simulink model "Nov12_RateModulated"  (R2019b)
settings: Solver=FixedStepAuto  StartTime=0.0  StopTime=10.0  FixedStep=1E-3  RelTol=1e-3
undefined symbols (not defined in the file): D0, D1, D10, D11, D12, D13, D2, D3, D4, D5, D6, D7, D8, D9, PTA0, PTA1, PTA2, PTB23, PTB9, PTC16, PTC17, PTC2, PTC3, PTC4, PTD0, PTD1, PTD2, PTD3
libraries: frdmk64flib x18
settings Model: PacingRate=0.100000  ExtModeTrigDuration=5  Creator=scotts24  LastModifiedBy=scotts24
settings DataIOCC: ReturnWorkspaceOutputs=off
settings OptimizationCC: PassReuseOutputArgsThreshold=0  MaxStackSize=64
settings DebuggingCC: ParameterTunabilityLossMsg=error  ArithmeticOperatorsInVariantConditions=warning
settings HardwareCC: ProdBitPerPointer=32  ProdBitPerSizeT=32  ProdBitPerPtrDiffT=32  ProdLargestAtomicInteger=Long  ProdLargestAtomicFloat=Double  ProdWordSize=32  ProdHWDeviceType=ARM Compatible->ARM Cortex  UseEmbeddedCoderFeatures=off
settings SFSimCC: SimUseLocalCustomCode=off  MATLABDynamicMemAlloc=off  CustomCodeUndefinedFunction=UseInterfaceOnly
settings RTWCC: SystemTargetFile=ert.tlc  HardwareBoard=NXP FRDM-K64F  TLCOptions="-aInlineSetEventsForThisBaseRateFcn=TLC_FALSE -aSuppressMultiTaskScheduler=TLC_FALSE  -aRateBasedStepFcn=0"  TemplateMakefile=ert_default_tmf  GenerateReport=on  RTWUseLocalCustomCode=off  Toolchain=GNU Tools for ARM Embedded Processors  LaunchReport=on
settings CodeAppCC: ForceParamTrailComments=on  OperatorAnnotations=on
settings ERTTargetCC: ERTCustomFileBanners=off  SupportContinuousTime=on  SupportNonInlinedSFcns=on  RemoveResetFunc=off  ModelStepFunctionPrototypeControlCompliant=off

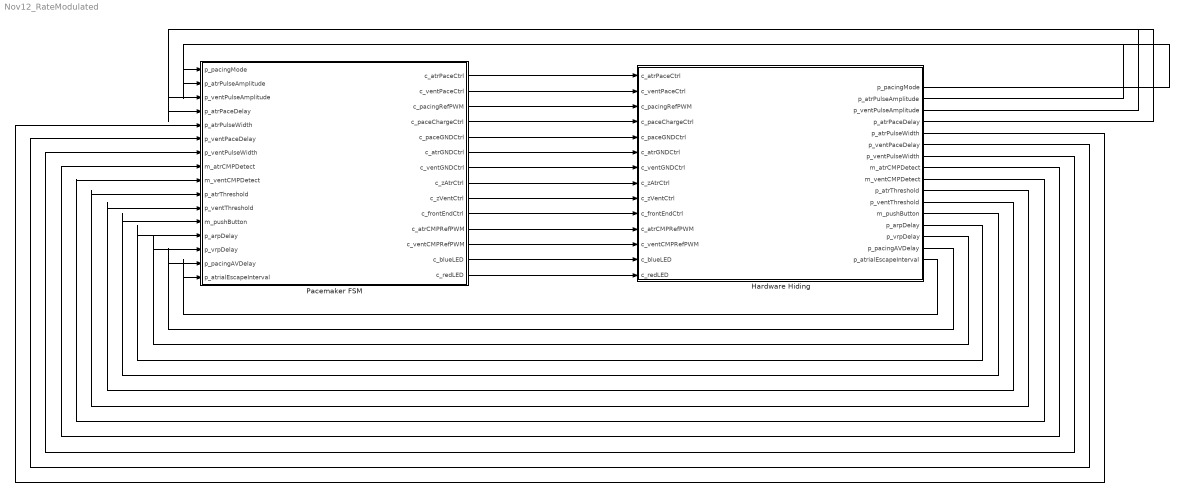
== system Nov12_RateModulated ==
  Hardware Hiding : Subsystem
  Pacemaker FSM : Stateflow chart  TreatAsAtomicUnit=on
  wires:
  Pacemaker FSM/9(c_zVentCtrl) -> Hardware Hiding/9(c_zVentCtrl)
  Pacemaker FSM/8(c_zAtrCtrl) -> Hardware Hiding/8(c_zAtrCtrl)
  Pacemaker FSM/7(c_ventGNDCtrl) -> Hardware Hiding/7(c_ventGNDCtrl)
  Pacemaker FSM/5(c_paceGNDCtrl) -> Hardware Hiding/5(c_paceGNDCtrl)
  Pacemaker FSM/6(c_atrGNDCtrl) -> Hardware Hiding/6(c_atrGNDCtrl)
  Pacemaker FSM/4(c_paceChargeCtrl) -> Hardware Hiding/4(c_paceChargeCtrl)
  Pacemaker FSM/3(c_pacingRefPWM) -> Hardware Hiding/3(c_pacingRefPWM)
  Pacemaker FSM/2(c_ventPaceCtrl) -> Hardware Hiding/2(c_ventPaceCtrl)
  Pacemaker FSM/1(c_atrPaceCtrl) -> Hardware Hiding/1(c_atrPaceCtrl)
  Pacemaker FSM/10(c_frontEndCtrl) -> Hardware Hiding/10(c_frontEndCtrl)
  Pacemaker FSM/11(c_atrCMPRefPWM) -> Hardware Hiding/11(c_atrCMPRefPWM)
  Pacemaker FSM/12(c_ventCMPRefPWM) -> Hardware Hiding/12(c_ventCMPRefPWM)
  Hardware Hiding/1(p_pacingMode) -> Pacemaker FSM/1(p_pacingMode)
  Hardware Hiding/2(p_atrPulseAmplitude) -> Pacemaker FSM/2(p_atrPulseAmplitude)
  Hardware Hiding/3(p_ventPulseAmplitude) -> Pacemaker FSM/3(p_ventPulseAmplitude)
  Hardware Hiding/4(p_atrPaceDelay) -> Pacemaker FSM/4(p_atrPaceDelay)
  Hardware Hiding/5(p_atrPulseWidth) -> Pacemaker FSM/5(p_atrPulseWidth)
  Hardware Hiding/6(p_ventPaceDelay) -> Pacemaker FSM/6(p_ventPaceDelay)
  Hardware Hiding/7(p_ventPulseWidth) -> Pacemaker FSM/7(p_ventPulseWidth)
  Hardware Hiding/8(m_atrCMPDetect) -> Pacemaker FSM/8(m_atrCMPDetect)
  Hardware Hiding/9(m_ventCMPDetect) -> Pacemaker FSM/9(m_ventCMPDetect)
  Hardware Hiding/10(p_atrThreshold) -> Pacemaker FSM/10(p_atrThreshold)
  Hardware Hiding/11(p_ventThreshold) -> Pacemaker FSM/11(p_ventThreshold)
  Hardware Hiding/12(m_pushButton) -> Pacemaker FSM/12(m_pushButton)
  Pacemaker FSM/13(c_blueLED) -> Hardware Hiding/13(c_blueLED)
  Pacemaker FSM/14(c_redLED) -> Hardware Hiding/14(c_redLED)
  Hardware Hiding/13(p_arpDelay) -> Pacemaker FSM/13(p_arpDelay)
  Hardware Hiding/14(p_vrpDelay) -> Pacemaker FSM/14(p_vrpDelay)
  Hardware Hiding/15(p_pacingAVDelay) -> Pacemaker FSM/15(p_pacingAVDelay)
  Hardware Hiding/16(p_atrialEscapeInterval) -> Pacemaker FSM/16(p_atrialEscapeInterval)

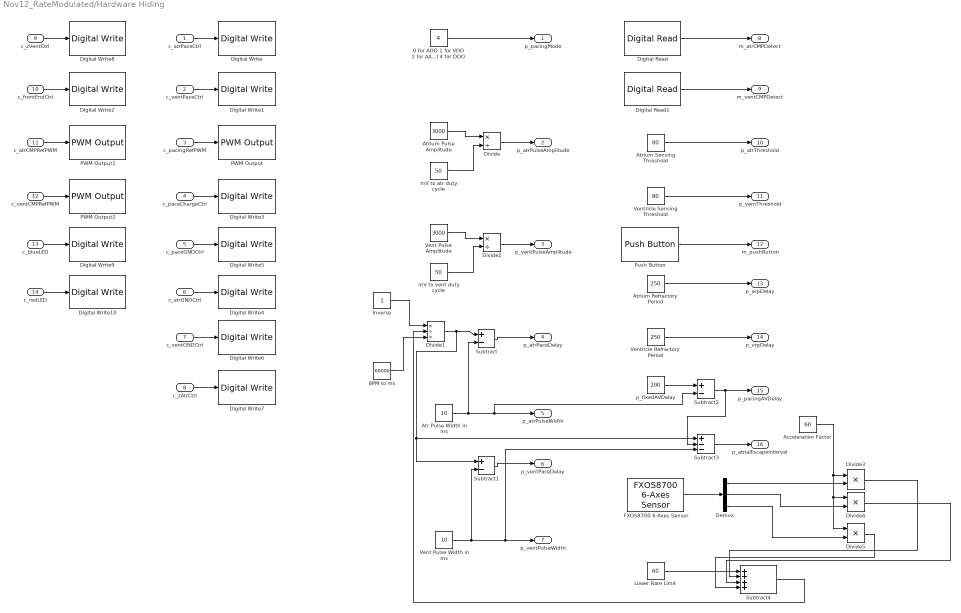
== system Nov12_RateModulated/Hardware Hiding ==
  c_atrPaceCtrl : Inport
  c_ventPaceCtrl : Inport  Port=2
  c_pacingRefPWM : Inport  Port=3
  c_paceChargeCtrl : Inport  Port=4
  c_paceGNDCtrl : Inport  Port=5
  c_atrGNDCtrl : Inport  Port=6
  c_ventGNDCtrl : Inport  Port=7
  c_zAtrCtrl : Inport  Port=8
  c_zVentCtrl : Inport  Port=9
  c_frontEndCtrl : Inport  Port=10
  c_atrCMPRefPWM : Inport  Port=11
  c_ventCMPRefPWM : Inport  Port=12
  c_blueLED : Inport  Port=13
  c_redLED : Inport  Port=14
  0 for AOO 1 for VOO 2 for AAI 3 for VVI 4 for DOO : Constant  Value=4  OutDataTypeStr=uint8
  Acceleration Factor : Constant  Value=60
  Atr Pulse Width in ms : Constant  Value=10  OutDataTypeStr=uint8
  Atrium Pulse Amplitude : Constant  Value=3000
  Atrium Refractory Period : Constant  Value=250  OutDataTypeStr=uint16
  Atrium Sensing Threshold : Constant  Value=80  OutDataTypeStr=uint8
  BPM to ms : Constant  Value=60000
  Demux : Demux  Outputs=3
  Digital Read : frdmk64flib/Digital Read  Whichpin=PTC16 (D0)  SampleTime=-1
      settings: SourceProductName=Simulink Coder Support Package for NXP FRDM-K64F Board
  Digital Read1 : frdmk64flib/Digital Read  Whichpin=PTC17 (D1)  SampleTime=-1
      settings: SourceProductName=Simulink Coder Support Package for NXP FRDM-K64F Board
  Digital Write : frdmk64flib/Digital Write  Whichpin=PTA0 (D8)
      settings: SourceProductName=Simulink Coder Support Package for NXP FRDM-K64F Board
  Digital Write1 : frdmk64flib/Digital Write  Whichpin=PTC4 (D9)
      settings: SourceProductName=Simulink Coder Support Package for NXP FRDM-K64F Board
  Digital Write10 : frdmk64flib/Digital Write  Whichpin=RED_LED
      settings: SourceProductName=Simulink Coder Support Package for NXP FRDM-K64F Board
  Digital Write2 : frdmk64flib/Digital Write  Whichpin=PTD1 (D13)
      settings: SourceProductName=Simulink Coder Support Package for NXP FRDM-K64F Board
  Digital Write3 : frdmk64flib/Digital Write  Whichpin=PTB9 (D2)
      settings: SourceProductName=Simulink Coder Support Package for NXP FRDM-K64F Board
  Digital Write4 : frdmk64flib/Digital Write  Whichpin=PTD2 (D11)
      settings: SourceProductName=Simulink Coder Support Package for NXP FRDM-K64F Board
  Digital Write5 : frdmk64flib/Digital Write  Whichpin=PTD0 (D10)
      settings: SourceProductName=Simulink Coder Support Package for NXP FRDM-K64F Board
  Digital Write6 : frdmk64flib/Digital Write  Whichpin=PTD3 (D12)
      settings: SourceProductName=Simulink Coder Support Package for NXP FRDM-K64F Board
  Digital Write7 : frdmk64flib/Digital Write  Whichpin=PTB23 (D4)
      settings: SourceProductName=Simulink Coder Support Package for NXP FRDM-K64F Board
  Digital Write8 : frdmk64flib/Digital Write  Whichpin=PTC3 (D7)
      settings: SourceProductName=Simulink Coder Support Package for NXP FRDM-K64F Board
  Digital Write9 : frdmk64flib/Digital Write  Whichpin=BLUE_LED
      settings: SourceProductName=Simulink Coder Support Package for NXP FRDM-K64F Board
  Divide : Product  Inputs=*/  OutDataTypeStr=uint8
  Divide1 : Product  Inputs=*/*  OutDataTypeStr=double
  Divide2 : Product  Inputs=*/  OutDataTypeStr=uint8
  Divide3 : Product  Inputs=**  OutDataTypeStr=double
  Divide4 : Product  Inputs=**  OutDataTypeStr=double
  Divide5 : Product  Inputs=**  OutDataTypeStr=double
  FXOS8700 6-Axes Sensor : frdmk64flib/FXOS8700 6-Axes Sensor  Activesensor=Accelerometer only  ODR=800Hz  HybridODR=400Hz  Accelfullrange=-4g to +4g  SampleTime=-1
      settings: SourceProductName=Simulink Coder Support Package for NXP FRDM-K64F Board
  Inverse : Constant
  Lower Rate Limit : Constant  Value=60
  PWM Output : frdmk64flib/PWM Output  Whichpin=PTA2 (D5)  InitialFrequency=2000  InitialDutyCycle=0
      settings: SourceProductName=Simulink Coder Support Package for NXP FRDM-K64F Board
  PWM Output1 : frdmk64flib/PWM Output  Whichpin=PTC2 (D6)  InitialFrequency=2000  InitialDutyCycle=0
      settings: SourceProductName=Simulink Coder Support Package for NXP FRDM-K64F Board
  PWM Output2 : frdmk64flib/PWM Output  Whichpin=PTA1 (D3)  InitialFrequency=2000  InitialDutyCycle=0
      settings: SourceProductName=Simulink Coder Support Package for NXP FRDM-K64F Board
  Push Button : frdmk64flib/Push Button  Whichswitch=SW2  SampleTime1=-1
      settings: SourceProductName=Simulink Coder Support Package for NXP FRDM-K64F Board
  Subtract : Sum  Inputs=+-  OutDataTypeStr=uint16
  Subtract1 : Sum  Inputs=+-  OutDataTypeStr=uint16
  Subtract2 : Sum  Inputs=+-  OutDataTypeStr=uint16
  Subtract3 : Sum  Inputs=+--  OutDataTypeStr=uint16
  Subtract4 : Sum  Inputs=++++  OutDataTypeStr=uint16
  Vent Pulse Amplitude : Constant  Value=3000
  Vent Pulse Width in ms : Constant  Value=10  OutDataTypeStr=uint8
  Ventricle Refractory Period : Constant  Value=250  OutDataTypeStr=uint16
  Ventricle Sensing Threshold : Constant  Value=80  OutDataTypeStr=uint8
  mV to atr duty cycle : Constant  Value=50
  mV to vent duty cycle : Constant  Value=50
  p_fixedAVDelay : Constant  Value=200
  p_pacingMode : Outport  VectorParamsAs1DForOutWhenUnconnected=off
  p_atrPulseAmplitude : Outport  Port=2  VectorParamsAs1DForOutWhenUnconnected=off
  p_ventPulseAmplitude : Outport  Port=3  VectorParamsAs1DForOutWhenUnconnected=off
  p_atrPaceDelay : Outport  Port=4  VectorParamsAs1DForOutWhenUnconnected=off
  p_atrPulseWidth : Outport  Port=5  VectorParamsAs1DForOutWhenUnconnected=off
  p_ventPaceDelay : Outport  Port=6  VectorParamsAs1DForOutWhenUnconnected=off
  p_ventPulseWidth : Outport  Port=7  VectorParamsAs1DForOutWhenUnconnected=off
  m_atrCMPDetect : Outport  Port=8
  m_ventCMPDetect : Outport  Port=9
  p_atrThreshold : Outport  Port=10  VectorParamsAs1DForOutWhenUnconnected=off
  p_ventThreshold : Outport  Port=11  VectorParamsAs1DForOutWhenUnconnected=off
  m_pushButton : Outport  Port=12
  p_arpDelay : Outport  Port=13  VectorParamsAs1DForOutWhenUnconnected=off
  p_vrpDelay : Outport  Port=14  VectorParamsAs1DForOutWhenUnconnected=off
  p_pacingAVDelay : Outport  Port=15  VectorParamsAs1DForOutWhenUnconnected=off
  p_atrialEscapeInterval : Outport  Port=16  VectorParamsAs1DForOutWhenUnconnected=off
  wires:
  c_atrPaceCtrl/1 -> Digital Write/1
  c_ventPaceCtrl/1 -> Digital Write1/1
  c_pacingRefPWM/1 -> PWM Output/1
  c_paceChargeCtrl/1 -> Digital Write3/1
  c_atrGNDCtrl/1 -> Digital Write4/1
  c_paceGNDCtrl/1 -> Digital Write5/1
  c_ventGNDCtrl/1 -> Digital Write6/1
  c_zAtrCtrl/1 -> Digital Write7/1
  c_zVentCtrl/1 -> Digital Write8/1
  0 for AOO 1 for VOO 2 for AAI 3 for VVI 4 for DOO/1 -> p_pacingMode/1
  Atrium Pulse Amplitude/1 -> Divide/1
  mV to atr duty cycle/1 -> Divide/2
  Divide/1 -> p_atrPulseAmplitude/1
  Subtract/1 -> p_atrPaceDelay/1
  mV to vent duty cycle/1 -> Divide2/2
  Vent Pulse Amplitude/1 -> Divide2/1
  Divide2/1 -> p_ventPulseAmplitude/1
  Atr Pulse Width in ms/1 -> Subtract/2, Subtract2/2, p_atrPulseWidth/1
  Vent Pulse Width in ms/1 -> Subtract1/2, Subtract3/3, p_ventPulseWidth/1
  Subtract1/1 -> p_ventPaceDelay/1
  Divide1/1 -> Subtract1/1, Subtract3/1, Subtract/1
  Digital Read/1 -> m_atrCMPDetect/1
  Digital Read1/1 -> m_ventCMPDetect/1
  BPM to ms/1 -> Divide1/3
  Inverse/1 -> Divide1/1
  c_frontEndCtrl/1 -> Digital Write2/1
  c_atrCMPRefPWM/1 -> PWM Output1/1
  Atrium Sensing Threshold/1 -> p_atrThreshold/1
  Ventricle Sensing Threshold/1 -> p_ventThreshold/1
  c_ventCMPRefPWM/1 -> PWM Output2/1
  Push Button/1 -> m_pushButton/1
  c_redLED/1 -> Digital Write10/1
  c_blueLED/1 -> Digital Write9/1
  Ventricle Refractory Period/1 -> p_vrpDelay/1
  Atrium Refractory Period/1 -> p_arpDelay/1
  p_fixedAVDelay/1 -> Subtract2/1
  Subtract2/1 -> Subtract3/2, p_pacingAVDelay/1
  Subtract3/1 -> p_atrialEscapeInterval/1
  FXOS8700 6-Axes Sensor/1 -> Demux/1
  Demux/2 -> Divide4/2
  Demux/3 -> Divide5/2
  Divide3/1 -> Subtract4/2
  Lower Rate Limit/1 -> Subtract4/1
  Acceleration Factor/1 -> Divide5/1, Divide4/1, Divide3/1
  Demux/1 -> Divide3/2
  Divide4/1 -> Subtract4/3
  Divide5/1 -> Subtract4/4
  Subtract4/1 -> Divide1/2

== stateflow chart Nov12_RateModulated/Pacemaker FSM ==
  note: In this state, we are allowing current to flow from C22
      | across the impendence of the atrium to C21 to generate an
      | artificial pace in the atrium. The LED is set to blue.
  note: In this state, we are allowing current to flow from C22
      | across the impendence of the ventricle to C21 to generate an
      | artificial pace in the ventricle. The LED is set to red.
  state A_PACING
    entry:
    c_paceChargeCtrl = false;
    c_paceGNDCtrl = true;
    c_ventPaceCtrl = false;
    c_ventGNDCtrl = false;
    c_zAtrCtrl = false;
    c_zVentCtrl = false;
    c_atrGNDCtrl = false;
    c_atrPaceCtrl = true;
    c_blueLED = true;
  state V_PACING
    entry:
    c_paceChargeCtrl = false;
    c_paceGNDCtrl = true;
    c_atrPaceCtrl = false;
    c_atrGNDCtrl = false;
    c_zAtrCtrl = false;
    c_zVentCtrl = false;
    c_ventGNDCtrl = false;
    c_ventPaceCtrl = true;
    c_redLED = true;
  note: Move from charging the C22 capacitor to pacing
      | the atrium after the delay atrPaceDelay which is the
      | time in between atrium paces depending on the BPM.
  note: Move from charging the C22 capacitor to pacing
      | the ventricle after the delay ventPaceDelay which is the
      | time in between ventricle paces depending on the BPM.
  note: Move from pacing the ventricle to charging the C22
      | capacitor after the delay ventPulseWidth which is the
      | programmed ventricle pulse width.
  note: Move from pacing the atrium to charging the C22
      | capacitor after the delay atrPulseWidth which is the
      | programmed atrium pulse width.
  state A_CHARGING
    entry:
    c_atrCMPRefPWM = p_atrThreshold;
    c_pacingRefPWM = p_atrPulseAmplitude;
    c_paceGNDCtrl = true;
    c_atrPaceCtrl = false;
    c_zAtrCtrl = false;
    c_zVentCtrl = false;
    c_ventPaceCtrl = false;
    c_ventGNDCtrl = false;
    c_atrGNDCtrl = true;
    c_paceChargeCtrl = true;
    c_blueLED = false;
  state V_CHARGING
    entry:
    c_ventCMPRefPWM = p_ventThreshold;
    c_pacingRefPWM = p_ventPulseAmplitude;
    c_paceGNDCtrl = true;
    c_ventPaceCtrl = false;
    c_zAtrCtrl = false;
    c_zVentCtrl = false;
    c_atrPaceCtrl = false;
    c_atrGNDCtrl = false;
    c_ventGNDCtrl = true;
    c_paceChargeCtrl = true;
    c_redLED = false;
  state INIT
    entry:
    c_frontEndCtrl = true;
    c_pacingRefPWM = 0;
    c_paceChargeCtrl = false;
    c_atrPaceCtrl = false;
    c_ventPaceCtrl = false;
    c_atrGNDCtrl = false;
    c_ventGNDCtrl = false;
    c_paceGNDCtrl = false;
    c_blueLED = false;
    c_redLED = false;
  note: True if the pacing mode is AOO, AAI, or DOO
  note: True if the pacing mode is VOO or VVI
  note: In this state, we are both charging the C22 capacitor,
      | and reversing current flow throug the ventricle in order
      | to create zero net charge. This is done by first
      | ensuring the patient is not directly connected to the
      | voltage supply by setting ventiPaceCtrl to false, which
      | opens the switch to prevent current flow from
      | C22 to C21.
  note: In this state, we are both charging the C22 capacitor,
      | and reversing current flow throug the atrium in order
      | to create zero net charge. This is done by first
      | ensuring the patient is not directly connected to the
      | voltage supply by setting atriPaceCtrl to false, which
      | opens the switch to prevent current flow from
      | C22 to C21.
  note: In this initial state, all switches are open and there is no current
      | flow in the system. The pacemaker then goes to the appropriate
      | atrium or ventricle charging states depending on which mode
      | is being implemented.
  note: This self-loop is used in sensing modes. Sensing does not begin until
      | after the atrium refractory period which is the atrDelay. When
      | a pace is sensed in the atrium, m_atrCMPDetect is set to true
      | and we stay in the charging state because we want to inhibit the next atrium
      | pace. Pushing the button will also satisfy this condition and inhibit a pace.
  note: This self-loop is used in sensing modes. Sensing does not begin until
      | after the ventricle refractory period which is the vtrDelay. When
      | a pace is sensed in the ventricle, m_ventCMPDetect is set to true
      | and we stay in the charging state because we want to inhibit the next ventricle
      | pace. Pushing the button will also satisfy this condition and inhibit a pace.
  V_CHARGING -> A_PACING [order 3] : [after(p_atrialEscapeInterval, msec) && p_pacingMode == 4]
  A_CHARGING -> V_PACING [order 3] : [after(p_pacingAVDelay, msec) && p_pacingMode == 4]
  A_PACING -> A_CHARGING : [after(p_atrPulseWidth, msec)]
  V_PACING -> V_CHARGING : [after(p_ventPulseWidth, msec)]
  A_CHARGING -> A_PACING [order 1] : [after(p_atrPaceDelay, msec)]
  V_CHARGING -> V_PACING [order 1] : [after(p_ventPaceDelay, msec)]
  (default) -> INIT
  INIT -> A_CHARGING [order 2] : [p_pacingMode == 0 || p_pacingMode == 2 || p_pacingMode == 4]
  INIT -> V_CHARGING [order 1] : [p_pacingMode == 1 || p_pacingMode == 3]
  V_CHARGING -> V_CHARGING [order 2] : [after(p_vrpDelay, msec) && p_pacingMode == 3 && m_ventCMPDetect == true || m_pushButton == true]
  A_CHARGING -> A_CHARGING [order 2] : [after(p_arpDelay, msec) && p_pacingMode == 2 && m_atrCMPDetect == true || m_pushButton == true]
  data: c_atrPaceCtrl output boolean; c_ventPaceCtrl output boolean; c_pacingRefPWM output uint8; c_paceChargeCtrl output boolean; c_paceGNDCtrl output boolean; c_atrGNDCtrl output boolean; c_ventGNDCtrl output boolean; c_zAtrCtrl output boolean; c_zVentCtrl output boolean; p_pacingMode input uint8; p_atrPulseAmplitude input uint8; p_ventPulseAmplitude input uint8; p_atrPaceDelay input uint16; p_atrPulseWidth input uint8; p_ventPaceDelay input uint16; p_ventPulseWidth input uint8; m_atrCMPDetect input boolean; m_ventCMPDetect input boolean; c_frontEndCtrl output boolean; c_atrCMPRefPWM output uint8; p_atrThreshold input uint8; p_ventThreshold input uint8; c_ventCMPRefPWM output uint8; m_pushButton input boolean; c_blueLED output boolean; c_redLED output boolean; p_arpDelay input uint16; p_vrpDelay input uint16; p_pacingAVDelay input uint16; p_atrialEscapeInterval input uint16
